simulink model "fixedliner"  (R2025a)
settings: Solver=ode4  StartTime=0.0  StopTime=0.5  FixedStep=0.0001  RelTol=1e-3
settings Model: Creator=Faheem  LastModifiedBy=Faheem

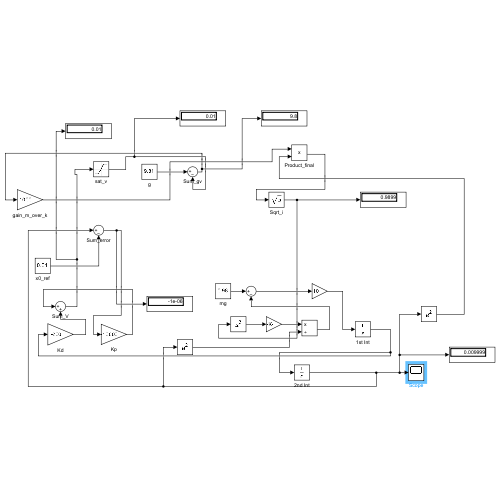
[thumbnail: Simulink's stored preview of the top-level diagram]
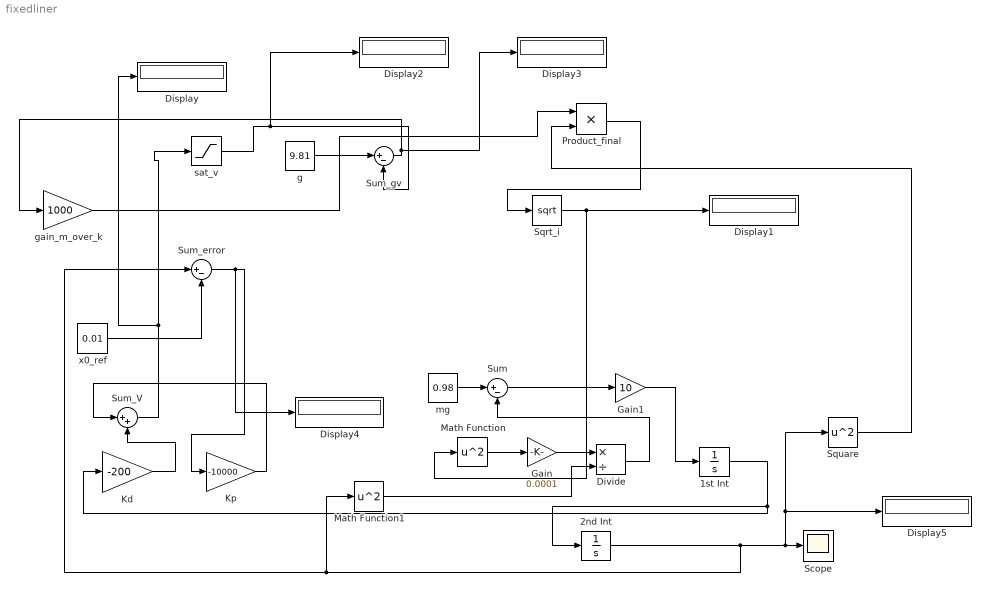
== system fixedliner ==
  1st Int : Integrator
  2nd Int : Integrator  InitialCondition=.015
  Display{,1..5} (6 alike) : Display
  Divide : Product  Inputs=*/
  Gain : Gain  Gain=0.0001
  Gain1 : Gain  Gain=10
  Kd : Gain  Gain=-200
  Kp : Gain  Gain=-10000
  Math Function : Math  Operator=square
  Math Function1 : Math  Operator=square
  Product_final : Product
  Scope : Scope
      settings: ActiveDisplayYMinimum=0.0093738750000000749  ActiveDisplayYMaximum=0.015625124999999993
  Sqrt_i : Sqrt
  Square : Math  Operator=square
  Sum : Sum  Inputs=|+-
  Sum_V : Sum  Inputs=|++
  Sum_error : Sum  Inputs=|+-
  Sum_gv : Sum  Inputs=|+-
  g : Constant  Value=9.81
  gain_m_over_k : Gain  Gain=1000
  mg : Constant  Value=0.98
  sat_v : Saturate  UpperLimit=9.3  LowerLimit=-1000
  x0_ref : Constant  Value=0.01
  wires:
  Divide/1 -> Sum/2
  Gain1/1 -> 1st Int/1
  Gain/1 -> Divide/1
  Math Function1/1 -> Divide/2
  1st Int/1 -> Kd/1, 2nd Int/1
  mg/1 -> Sum/1
  Sum/1 -> Gain1/1
  2nd Int/1 -> Scope/1, Display5/1, Square/1, Math Function1/1, Sum_error/1
  Math Function/1 -> Gain/1
  x0_ref/1 -> Sum_error/2
  Sum_error/1 -> Display4/1, Kp/1
  Kp/1 -> Sum_V/1
  Kd/1 -> Sum_V/2
  Sum_V/1 -> Display/1, sat_v/1
  g/1 -> Sum_gv/1
  sat_v/1 -> Display2/1, Sum_gv/2
  Sum_gv/1 -> Display3/1, gain_m_over_k/1
  gain_m_over_k/1 -> Product_final/1
  Product_final/1 -> Sqrt_i/1
  Sqrt_i/1 -> Display1/1, Math Function/1
  Square/1 -> Product_final/2
